simulink model "glideslopecontroller"  (R2021a)
settings: Solver=VariableStepAuto  StartTime=0.0  StopTime=10.0  RelTol=1e-3
settings Model: Creator=ba23m  LastModifiedBy=ba23m

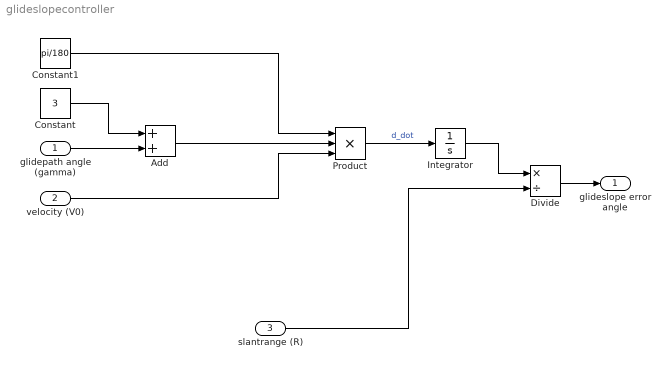
== system glideslopecontroller ==
  glidepath angle (gamma) : Inport
  velocity (V0) : Inport  Port=2
  slantrange (R) : Inport  Port=3
  Add : Sum
  Constant : Constant  Value=3
  Constant1 : Constant  Value=pi/180
  Divide : Product  Inputs=*/
  Integrator : Integrator
  Product : Product  Inputs=3
  glideslope error angle : Outport
  wires:
  Constant/1 -> Add/1
  glidepath angle (gamma)/1 -> Add/2
  Constant1/1 -> Product/1
  Add/1 -> Product/2
  velocity (V0)/1 -> Product/3
  Product/1 -> Integrator/1  "d_dot"
  Integrator/1 -> Divide/1
  slantrange (R)/1 -> Divide/2
  Divide/1 -> glideslope error angle/1
